simulink model "MultiFOC"  (R2023b)
settings: Solver=FixedStepDiscrete  StartTime=0.0  StopTime=10.0  RelTol=1e-3
undefined symbols (not defined in the file): D1, D2, D3, D4, P
settings Model: DataDictionary=EmbeddedBoardDD.sldd  Creator=mfussi  LastModifiedBy=mfussi
settings OptimizationCC: DefaultParameterBehavior=Inlined  EnhancedBackFolding=on  PassReuseOutputArgsAs=Individual arguments  ZeroExternalMemoryAtStartup=off  ZeroInternalMemoryAtStartup=off  OptimizeBlockOrder=speed  DifferentSizesBufferReuse=on  OptimizationCustomize=off  EfficientTunableParamExpr=on
settings DebuggingCC: ParameterTunabilityLossMsg=error
settings SFSimCC: MATLABDynamicMemAlloc=off
settings RTWCC: Description=Embedded Coder  SystemTargetFile=ert.tlc  TemplateMakefile=ert_default_tmf
settings CodeAppCC: ForceParamTrailComments=on  IgnoreCustomStorageClasses=off  OperatorAnnotations=on  SimulinkDataObjDesc=on  SFDataObjDesc=on  InsertBlockDesc=on
settings ERTTargetCC: TargetLangStandard=C99 (ISO)  GenerateSampleERTMain=on  InlinedParameterPlacement=NonHierarchical  ERTCustomFileTemplate=example_file_process.tlc

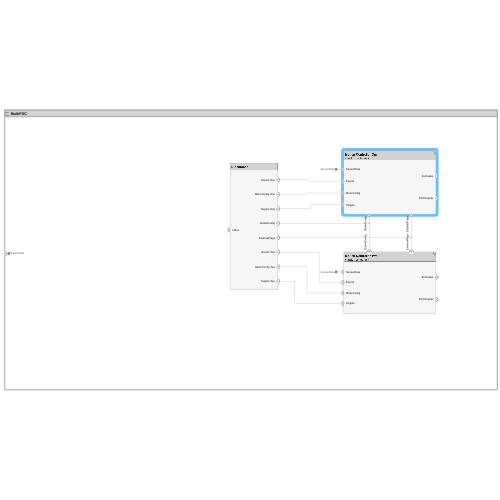
[thumbnail: Simulink's stored preview of the top-level diagram]
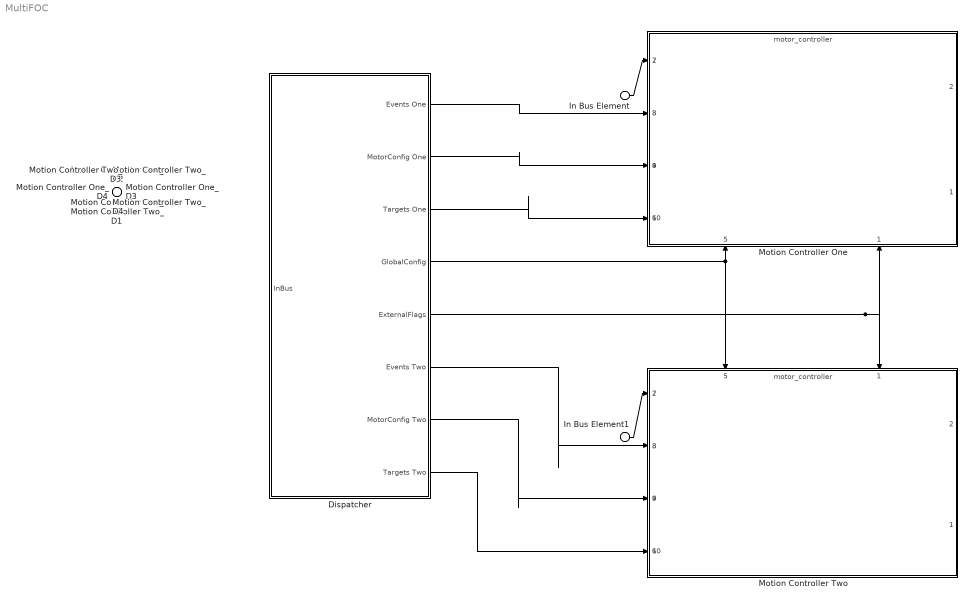
== system MultiFOC ==
  In Bus Element : Inport  PortName=SensorData
  In Bus Element1 : Inport  PortName=SensorData
  Motion Controller One_D1 : Inport  Port=2  OutputFunctionCall=on
  Motion Controller One_D2 : Inport  Port=3  OutputFunctionCall=on
  Motion Controller One_D3 : Inport  Port=4  OutputFunctionCall=on
  Motion Controller One_D4 : Inport  Port=5  OutputFunctionCall=on
  Motion Controller Two_D1 : Inport  Port=6  OutputFunctionCall=on
  Motion Controller Two_D2 : Inport  Port=7  OutputFunctionCall=on
  Motion Controller Two_D3 : Inport  Port=8  OutputFunctionCall=on
  Motion Controller Two_D4 : Inport  Port=9  OutputFunctionCall=on
  Dispatcher : Subsystem
      settings: PortSchema="{\"entries\":[{\"content\":{\"headerSize\":26,\"margin\":15,\"minimumSpacing\":25,\"sides\":[{\"content\":{\"connectorIds\":[\"In1\"]},\"type\":\"ConnectorPlacement.EquallySpacedRectSide\",\"uuid\":\"1f7f87e2-1f9b-4f9b-81b4-f2a20d6d1e5a\"},{\"content\":{\"connectorIds\":[\"Out1\",\"Out3\",\"Out5\",\"Out4\",\"Out2\",\"Out6\",\"Out7\",\"Out8\"],\"side\":\"RIGHT\"},\"type\":\"ConnectorPlacement.EquallySpacedRectSide\",\"uuid\":\"8d2207c1-aa11-40f1-ac28-76b1f5a19d47\"},{\"content\":{\"side\":\"TOP\"},\"type\":\"ConnectorPlacement.EquallySpacedRectSide\",\"uuid\":\"c1e2b4f8-7873-4bf9-83d5-cc49fa0f92db\"}]},\"type\":\"ConnectorPlacement.EquallySpacedConnector\",\"uuid\":\"6bf0649d-fad0-4b80-86c4-bbc9d6571a2e\"}],\"packageUris\":[\"http://schema.mathworks.com/mf0/Connector/R2020b\"],\"version\":\"1.0\"}"
  Motion Controller One : ModelReference  ModelNameDialog=motor_controller.slx  SimulationMode=Normal  ScheduleRates=on  CachedPortDiscreteRates=[1.1428571428571438E-6;3.65714285714286E-5;0.001;0.01]  ModelEventPortInfo=P:D1[1.1428571428571438E-6][0][0],P:D2[3.65714285714286E-5][0][0],P:D3[0.001][0][0],P:D4[0.01][0][0]  ModelReferenceVersion=2.0
      settings: PortSchema="{\"entries\":[{\"content\":{\"headerSize\":38,\"margin\":15,\"minimumSpacing\":25,\"sides\":[{\"content\":{\"connectorIds\":[\"In2\",\"In3\",\"In4\",\"In6\"]},\"type\":\"ConnectorPlacement.EquallySpacedRectSide\",\"uuid\":\"226473d0-e073-493e-8c8e-6196a9f9e149\"},{\"content\":{\"connectorIds\":[\"Out2\",\"Out1\"],\"side\":\"RIGHT\"},\"type\":\"ConnectorPlacement.EquallySpacedRectSide\",\"uuid\":\"7073cbea-f16a-4377-b922-078090dcef9d\"},{\"content\":{\"side\":\"TOP\"},\"type\":\"ConnectorPlacement.EquallySpacedRectSide\",\"uuid\":\"c3ec4a69-cf36-47e0-a219-ce59208b03e4\"},{\"content\":{\"connectorIds\":[\"In5\",\"In1\"],\"side\":\"BOTTOM\"},\"type\":\"ConnectorPlacement.EquallySpacedRectSide\",\"uuid\":\"388c9924-2125-4d02-93a5-948073c77c6f\"},{\"content\":{\"connectorIds\":[\"In7\",\"In8\",\"In9\",\"In10\"],\"side\":\"HIDDEN\"},\"type\":\"ConnectorPlacement.EquallySpacedRectSide\",\"uuid\":\"6609e07d-5850-401a-a8c3-c851c3e84a03\"}]},\"type\":\"ConnectorPlacement.EquallySpacedConnector\",\"uuid\":\"48f02d1d-6e21-4533-87ad-ecd8a4ee6157\"}],\"packageUris\":[\"http://schema.mathworks.com/mf0/Connector/R2020b\"],\"version\":\"1.0\"}"
  Motion Controller Two : ModelReference  ModelNameDialog=motor_controller.slx  SimulationMode=Normal  ScheduleRates=on  CachedPortDiscreteRates=[1.1428571428571438E-6;3.65714285714286E-5;0.001;0.01]  ModelEventPortInfo=P:D1[1.1428571428571438E-6][0][0],P:D2[3.65714285714286E-5][0][0],P:D3[0.001][0][0],P:D4[0.01][0][0]  ModelReferenceVersion=2.0
      settings: PortSchema="{\"entries\":[{\"content\":{\"headerSize\":38,\"margin\":15,\"minimumSpacing\":25,\"sides\":[{\"content\":{\"connectorIds\":[\"In2\",\"In3\",\"In4\",\"In6\"]},\"type\":\"ConnectorPlacement.EquallySpacedRectSide\",\"uuid\":\"226473d0-e073-493e-8c8e-6196a9f9e149\"},{\"content\":{\"connectorIds\":[\"Out2\",\"Out1\"],\"side\":\"RIGHT\"},\"type\":\"ConnectorPlacement.EquallySpacedRectSide\",\"uuid\":\"7073cbea-f16a-4377-b922-078090dcef9d\"},{\"content\":{\"connectorIds\":[\"In5\",\"In1\"],\"side\":\"TOP\"},\"type\":\"ConnectorPlacement.EquallySpacedRectSide\",\"uuid\":\"c3ec4a69-cf36-47e0-a219-ce59208b03e4\"},{\"content\":{\"connectorIds\":[\"In7\",\"In8\",\"In9\",\"In10\"],\"side\":\"HIDDEN\"},\"type\":\"ConnectorPlacement.EquallySpacedRectSide\",\"uuid\":\"6609e07d-5850-401a-a8c3-c851c3e84a03\"}]},\"type\":\"ConnectorPlacement.EquallySpacedConnector\",\"uuid\":\"48f02d1d-6e21-4533-87ad-ecd8a4ee6157\"}],\"packageUris\":[\"http://schema.mathworks.com/mf0/Connector/R2020b\"],\"version\":\"1.0\"}"
  wires:
  Dispatcher/1(Events One) -> Motion Controller One/3
  In Bus Element/1 -> Motion Controller One/2
  Dispatcher/3(MotorConfig One) -> Motion Controller One/4
  Dispatcher/5(Targets One) -> Motion Controller One/6
  Dispatcher/2(ExternalFlags) -> Motion Controller Two/1, Motion Controller One/1
  Dispatcher/4(GlobalConfig) -> Motion Controller Two/5, Motion Controller One/5
  Dispatcher/7(MotorConfig Two) -> Motion Controller Two/4
  Dispatcher/6(Events Two) -> Motion Controller Two/3
  In Bus Element1/1 -> Motion Controller Two/2
  Dispatcher/8(Targets Two) -> Motion Controller Two/6

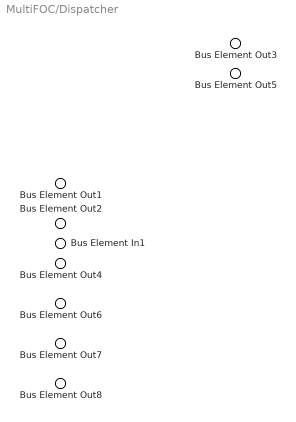
== system MultiFOC/Dispatcher ==
  Bus Element In1 : Inport  PortName=InBus
  Bus Element Out5 : Outport  PortName=Events One
  Bus Element Out1 : Outport  Port=2  PortName=ExternalFlags
  Bus Element Out3 : Outport  Port=3  PortName=MotorConfig One
  Bus Element Out2 : Outport  Port=4  PortName=GlobalConfig
  Bus Element Out4 : Outport  Port=5  PortName=Targets One
  Bus Element Out6 : Outport  Port=6  PortName=Events Two
  Bus Element Out7 : Outport  Port=7  PortName=MotorConfig Two
  Bus Element Out8 : Outport  Port=8  PortName=Targets Two
